simulink model "MinSegMega_Demo_V3"  (R2013a)
settings: Solver=FixedStepDiscrete  SolverMode=SingleTasking  StartTime=0.0  StopTime=inf  FixedStep=.1  RelTol=1e-3
libraries: arduinolib x10, MinSegLibrary_MinSegMega x2
settings Model: SimulationMode=external  ExtModeTrigDuration=2  Creator=Alec  LastModifiedBy=hurstj
settings OptimizationCC: ExpressionDepthLimit=2147483647  OptimizeModelRefInitCode=on  LifeSpan=1
settings DebuggingCC: SolverPrmCheckMsg=none  StrictBusMsg=Warning
settings HardwareCC: ProdBitPerInt=16  ProdBitPerPointer=8  ProdIntDivRoundTo=Zero  ProdEndianess=LittleEndian  ProdWordSize=8  ProdHWDeviceType=Atmel->AVR
settings RTWCC: SystemTargetFile=realtime.tlc  GenerateMakefile=off  TemplateMakefile=realtime.tmf  Description=Real-Time Toolbox  RTWVerbose=off  ProcessScript=realtime_make_rtw_hook
settings CodeAppCC: CustomSymbolStrType=$N$R$M  InternalIdentifier=Classic
settings STFCustomTargetCC: TargetLibSuffix=.a  GenerateSampleERTMain=on  ERTCustomFileBanners=on  SupportNonInlinedSFcns=off  SupportVariableSizeSignals=on  MATLABClassNameForMDSCustomization=Simulink.SoftwareTarget.ERTCustomization  SystemTargetFile=realtime.tlc
settings ERTTargetCC: ParMdlRefBuildCompliant=off  CompOptLevelCompliant=off  ConcurrentExecutionCompliant=off  CombineOutputUpdateFcns=off  ERTFirstTimeCompliant=off  SupportContinuousTime=on  SupportVariableSizeSignals=on  ModelStepFunctionPrototypeControlCompliant=off  CPPClassGenCompliant=off  ExtMode=on  ExtModeTransport=3  ExtModeMexFile=ext_serial_win32_comm  ExtModeMexArgs=0 66 115200  ERTSrcFileBannerTemplate=realtime_code_template.cgt  ERTHdrFileBannerTemplate=realtime_code_template.cgt  ERTDataSrcFileTemplate=realtime_code_template.cgt  ERTDataHdrFileTemplate=realtime_code_template.cgt  ERTCustomFileTemplate=realtime_file_process.tlc

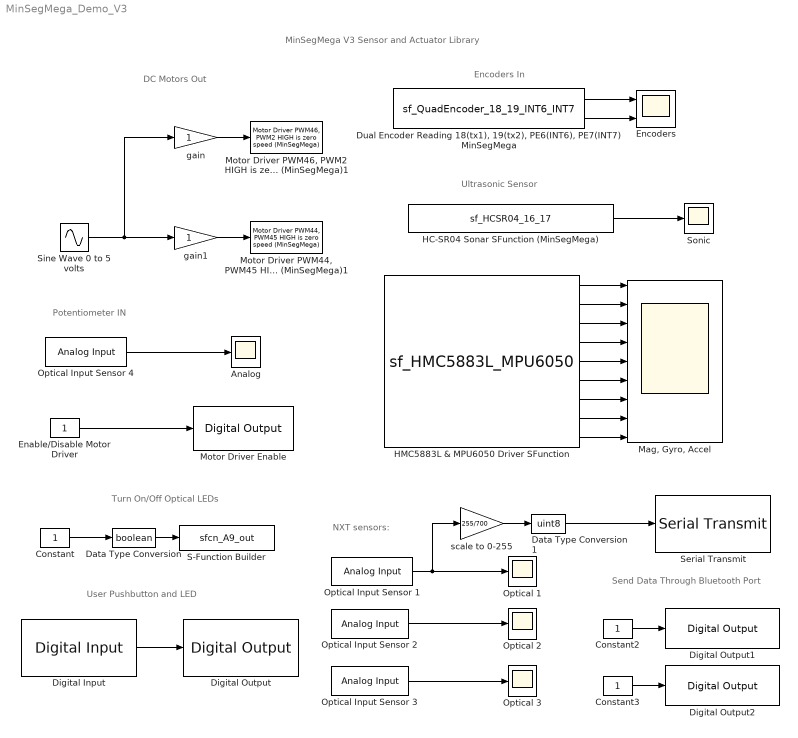
== system MinSegMega_Demo_V3 ==
  note: Turn On/Off Optical LEDs
  note: Send Data Through Bluetooth Port
  note: Potentiometer IN
  note: DC Motors Out
  note: Encoders In
  note: NXT sensors:
  note: User Pushbutton and LED
  note: Ultrasonic Sensor
  note: MinSegMega V3 Sensor and Actuator Library
  Analog : Scope
      settings: TimeRange=30  YMin=250  YMax=850  SaveName=ScopeData6
  Constant : Constant  SampleTime=-1
  Constant2 : Constant  SampleTime=-1
  Constant3 : Constant  SampleTime=-1
  Data Type Conversion : DataTypeConversion  OutDataTypeStr=boolean
  Data Type Conversion1 : DataTypeConversion  OutDataTypeStr=uint8
  Digital Input : arduinolib/Digital Input  pinNumber=53  sampleTime=-1
  Digital Output : arduinolib/Digital Output  pinNumber=49
  Digital Output1 : arduinolib/Digital Output  pinNumber=25
  Digital Output2 : arduinolib/Digital Output  pinNumber=48
  "Dual Encoder Reading 18(tx1), 19(tx2), PE6(INT6), PE7(INT7) MinSegMega " : S-Function  InitFcn=try, set_param(gcb,'FunctionName','sf_QuadEncoder_18_19_INT6_INT7'), end  FunctionName=sf_QuadEncoder_18_19_INT6_INT7  Parameters=uint8([0 1]),uint8([18 6]),uint8([19 7])  SFunctionModules=sf_QuadEncoder_18_19_INT6_INT7_wrapper  EnableBusSupport=off  mask(S-Function Builder){}
      mask init:
      | val = [[.9  0.75 0.75 1 1 .9 .9 1]',[1 1 0.75 0.75 .9 .9 1 .9]'];try , sys = get_param(gcb,'SfunBuilderFcnName');if isempty(sys), sys = get_param(gcb,'FunctionName'); end,catch, sys = get_param(gcb,'FunctionName'); end
      settings: CopyFcn=set_param(gcbh,'LinkStatus','none')  PreSaveFcn=try, set_param(gcb,'FunctionName','sf_QuadEncoder_18_19_INT6_INT7'), end  OpenFcn=sfunctionwizard(gcbh)
      mask Display: plot(val(:,1),val(:,2)),disp(sys), port_label('output',1,'pos1'), port_label('output',2,'pos2')
  Enable/Disable Motor Driver : Constant  SampleTime=-1
  Encoders : Scope  NumInputPorts=2
      settings: TimeRange=10  YMin=7750~-1  YMax=10250~1
  HC-SR04 Sonar SFunction (MinSegMega) : S-Function  InitFcn=try, set_param(gcb,'FunctionName','sf_HCSR04_16_17'), end  FunctionName=sf_HCSR04_16_17  SFunctionModules=sf_HCSR04_16_17_wrapper  EnableBusSupport=off  mask(S-Function Builder){}
      mask help: Simulink:masks:SFunctionBuilder_MD
      mask init: same as MinSegMega_Demo_V3/Dual Encoder Reading 18(tx1), 19(tx2), PE6(INT6), PE7(INT7) MinSegMega 
      settings: CopyFcn=set_param(gcbh,'LinkStatus','none')  PreSaveFcn=try, set_param(gcb,'FunctionName','sf_HCSR04_16_17'), end  OpenFcn=sfunctionwizard(gcbh)
      mask Display:
      | plot(val(:,1),val(:,2))
      | disp(sys)
      | port_label('output',1,'distance_cm')
  HMC5883L & MPU6050 Driver SFunction : S-Function  InitFcn=try, set_param(gcb,'FunctionName','sf_HMC5883L_MPU6050'), end  FunctionName=sf_HMC5883L_MPU6050  SFunctionModules=sf_HMC5883L_MPU6050_wrapper  EnableBusSupport=off  mask(S-Function Builder){}
      mask help: Simulink:masks:SFunctionBuilder_MD
      mask init: same as MinSegMega_Demo_V3/Dual Encoder Reading 18(tx1), 19(tx2), PE6(INT6), PE7(INT7) MinSegMega 
      settings: CopyFcn=set_param(gcbh,'LinkStatus','none')  PreSaveFcn=try, set_param(gcb,'FunctionName','sf_HMC5883L_MPU6050'), end  OpenFcn=sfunctionwizard(gcbh)
      mask Display:
      | plot(val(:,1),val(:,2))
      | disp(sys)
      | port_label('output',1,'x_mag')
      | port_label('output',2,'y_mag')
      | port_label('output',3,'z_mag')
      | port_label('output',4,'x_vel')
      | port_label('output',5,'y_vel')
      | port_label('output',6,'z_vel')
      | port_label('output',7,'x_acc')
      | port_label('output',8,'y_acc')
      | port_label('output',9,'z_acc')
  "Mag, Gyro, Accel" : Scope  NumInputPorts=9
      settings: TimeRange=10  YMin=-600~1050~-100~-40000~-25000~-40000~-3000~-10000~11000  YMax=-250~1400~150~40000~20000~30000~8000~12500~20000
  Motor Driver Enable : arduinolib/Digital Output  pinNumber=42
  "Motor Driver PWM44, PWM45 HIGH is zero speed (MinSegMega)1" : MinSegLibrary_MinSegMega/Motor Driver PWM44, PWM45 HIGH is zero speed (MinSegMega)
  "Motor Driver PWM46, PWM2 HIGH is zero speed (MinSegMega)1" : MinSegLibrary_MinSegMega/Motor Driver PWM46, PWM2 HIGH is zero speed (MinSegMega)
  Optical 1 : Scope
      settings: TimeRange=30  YMin=450  YMax=775  SaveName=ScopeData4
  Optical 2 : Scope
      settings: TimeRange=30  YMin=325  YMax=625  SaveName=ScopeData3
  Optical 3 : Scope
      settings: TimeRange=30  YMin=300  YMax=800  SaveName=ScopeData2
  Optical Input Sensor 1 : arduinolib/Analog Input  pinNumber=10  sampleTime=-1
  Optical Input Sensor 2 : arduinolib/Analog Input  pinNumber=11  sampleTime=-1
  Optical Input Sensor 3 : arduinolib/Analog Input  pinNumber=7  sampleTime=-1
  Optical Input Sensor 4 : arduinolib/Analog Input  pinNumber=13  sampleTime=-1
  S-Function Builder : S-Function  InitFcn=try, set_param(gcb,'FunctionName','sfcn_A9_out'), end  FunctionName=sfcn_A9_out  Parameters=uint8(9)  SFunctionModules=sfcn_A9_out_wrapper  EnableBusSupport=off  mask(S-Function Builder){}
      mask init: same as MinSegMega_Demo_V3/Dual Encoder Reading 18(tx1), 19(tx2), PE6(INT6), PE7(INT7) MinSegMega 
      settings: CopyFcn=set_param(gcbh,'LinkStatus','none')  PreSaveFcn=try, set_param(gcb,'FunctionName','sfcn_A9_out'), end  OpenFcn=sfunctionwizard(gcbh)
      mask Display: plot(val(:,1),val(:,2)),disp(sys), port_label('input',1,'in')
  Serial Transmit : arduinolib/Serial Transmit  portNumber=3
  Sine Wave 0 to 5 volts : Sin  SineType=Sample based  Amplitude=5  Frequency=50*2*pi  Samples=30  SampleTime=.1
  Sonic : Scope
      settings: TimeRange=30  YMin=0  YMax=55  SaveName=ScopeData7
  gain : Gain  OutDataTypeStr=int16
  gain1 : Gain  OutDataTypeStr=int16
  scale to 0-255 : Gain  Gain=255/700  OutDataTypeStr=int16
  wires:
  gain/1 -> "Motor Driver PWM46, PWM2 HIGH is zero speed (MinSegMega)1"/1
  Sine Wave 0 to 5 volts/1 -> gain1/1, gain/1
  gain1/1 -> "Motor Driver PWM44, PWM45 HIGH is zero speed (MinSegMega)1"/1
  "Dual Encoder Reading 18(tx1), 19(tx2), PE6(INT6), PE7(INT7) MinSegMega "/1 -> Encoders/1
  "Dual Encoder Reading 18(tx1), 19(tx2), PE6(INT6), PE7(INT7) MinSegMega "/2 -> Encoders/2
  Optical Input Sensor 1/1 -> scale to 0-255/1, Optical 1/1
  Constant/1 -> Data Type Conversion/1
  HMC5883L & MPU6050 Driver SFunction/1 -> "Mag, Gyro, Accel"/1
  HMC5883L & MPU6050 Driver SFunction/2 -> "Mag, Gyro, Accel"/2
  HMC5883L & MPU6050 Driver SFunction/3 -> "Mag, Gyro, Accel"/3
  HMC5883L & MPU6050 Driver SFunction/4 -> "Mag, Gyro, Accel"/4
  HMC5883L & MPU6050 Driver SFunction/5 -> "Mag, Gyro, Accel"/5
  HMC5883L & MPU6050 Driver SFunction/6 -> "Mag, Gyro, Accel"/6
  HMC5883L & MPU6050 Driver SFunction/7 -> "Mag, Gyro, Accel"/7
  HMC5883L & MPU6050 Driver SFunction/8 -> "Mag, Gyro, Accel"/8
  HMC5883L & MPU6050 Driver SFunction/9 -> "Mag, Gyro, Accel"/9
  scale to 0-255/1 -> Data Type Conversion1/1
  Data Type Conversion1/1 -> Serial Transmit/1
  Optical Input Sensor 2/1 -> Optical 2/1
  Optical Input Sensor 4/1 -> Analog/1
  Data Type Conversion/1 -> S-Function Builder/1
  Optical Input Sensor 3/1 -> Optical 3/1
  Digital Input/1 -> Digital Output/1
  Constant2/1 -> Digital Output1/1
  Constant3/1 -> Digital Output2/1
  HC-SR04 Sonar SFunction (MinSegMega)/1 -> Sonic/1
  Enable/Disable Motor Driver/1 -> Motor Driver Enable/1
